simulink model "ModeStatAndRsp"  (R2018b)
settings: Solver=FixedStepDiscrete  StartTime=0.0  StopTime=10.0  FixedStep=0.01  RelTol=1e-3
undefined symbols (not defined in the file): c_RecvL, c_RecvLR, c_RecvR, IfVeSMSeStNumConfig, KeSMSbMdChime2Enable_Val, KeSMSbSRSPosNumConfig_Val, KeSMSuChmReqDurnTm_Val, KeSMSuChmReqIntlTm_Val, KeSMSuRspStatHldTm_Val, MdRspLocal1, MdTp1, ModeNum, PowerMode1, SrcReqTp1, srsconvert
libraries: RspLib x47, simulink x1
(part 8 of 8)

== stateflow chart ModeStatAndRsp/ModeStatAndRsp_Runnable_sys/Subsystem1/Subsystem/Chart ==
  state OffState
    note: /*<REQ_MSM_228>*/
  state SeatBusyChk [function]
    (default) -> (junction 431)
    (junction 431) -> (junction 606) [order 1] : [is6s||is4s]
    (junction 606) -> (junction 777) [order 1] : [is4s]
    (junction 777) -> (junction 779) : {
        | EZEStBsy=1;
        | EZQStBsy=1;
        | LugLStBsy=1;
        | LugRStBsy=1;
        | INTMBsy=1;
        | FamlyLBsy=1;
        | FamlyRBsy=1;
        | INTMRBsy=1;
        | }
    (junction 431) -> (junction 495) [order 2]
    (junction 606) -> (junction 620) [order 2]
    (junction 495) -> (junction 504) [order 1] : [EZQ_En ||VIPL_En||VIPR_En||RecoveryL_En||RecoveryR_En||LugL_En||LugR_En||INTM_En||FAMLY_L_En||FAMLY_R_En||INTMR_En]
    (junction 620) -> (junction 631) [order 1] : [EZQ_En ||VIPL_En||VIPR_En||RecoveryL_En||RecoveryR_En||LugL_En||LugR_En||INTM_En||FAMLY_L_En||FAMLY_R_En||INTMR_En]
    (junction 495) -> (junction 508) [order 2] : {EZEStBsy=0;}
    (junction 504) -> (junction 506) : {EZEStBsy=1;}
    (junction 620) -> (junction 628) [order 2] : {EZEStBsy=0;}
    (junction 631) -> (junction 632) : {EZEStBsy=1;}
    (junction 506) -> (junction 508)
    (junction 632) -> (junction 628)
    (junction 508) -> (junction 511)
    (junction 628) -> (junction 609)
    (junction 609) -> (junction 621) [order 1] : [EZE_En ||VIPL_En||VIPR_En||RecoveryL_En||RecoveryR_En||LugL_En||LugR_En||INTM_En||FAMLY_L_En||FAMLY_R_En||INTMR_En]
    (junction 511) -> (junction 513) [order 1] : [EZE_En ||VIPL_En||VIPR_En||RecoveryL_En||RecoveryR_En||LugL_En||LugR_En||INTM_En||FAMLY_L_En||FAMLY_R_En||INTMR_En]
    (junction 511) -> (junction 517) [order 2] : {EZQStBsy=0;}
    (junction 513) -> (junction 515) : {EZQStBsy=1;}
    (junction 609) -> (junction 624) [order 2] : {EZQStBsy=0;}
    (junction 621) -> (junction 622) : {EZQStBsy=1;}
    (junction 515) -> (junction 517)
    (junction 622) -> (junction 624)
    (junction 517) -> (junction 520)
    (junction 624) -> (junction 619)
    (junction 619) -> (junction 615) [order 1] : [EZE_En||EZQ_En ||RecoveryL_En||LugL_En||INTM_En||FAMLY_L_En||FAMLY_R_En||LugR_En||INTMR_En]
    (junction 520) -> (junction 522) [order 1] : [EZE_En||EZQ_En ||RecoveryL_En||LugL_En||LugR_En||INTM_En||FAMLY_L_En||FAMLY_R_En||INTMR_En]
    (junction 520) -> (junction 526) [order 2] : {VIPLStBsy = 0;}
    (junction 522) -> (junction 524) : {VIPLStBsy = 1;}
    (junction 619) -> (junction 623) [order 2] : {VIPLStBsy = 0;}
    (junction 615) -> (junction 614) : {VIPLStBsy = 1;}
    (junction 524) -> (junction 526)
    (junction 614) -> (junction 623)
    (junction 526) -> (junction 529)
    (junction 623) -> (junction 633)
    (junction 779) -> (junction 781) [order 1] : [LyL_En ||RecoveryL_En||LgrstOpenL_En||LgrstCloseL_En]
    (junction 779) -> (junction 785) [order 2] : {VIPLStBsy = 0;}
    (junction 781) -> (junction 783) : {VIPLStBsy = 1;}
    (junction 529) -> (junction 531) [order 1] : [EZE_En||EZQ_En ||RecoveryR_En||LugL_En||LugR_En||INTM_En||FAMLY_L_En||FAMLY_R_En||INTMR_En]
    (junction 633) -> (junction 608) [order 1] : [EZE_En||EZQ_En ||RecoveryR_En||LugR_En||INTM_En||FAMLY_L_En||FAMLY_R_En||LugL_En||INTMR_En]
    (junction 529) -> (junction 535) [order 2] : {VIPRStBsy = 0;}
    (junction 531) -> (junction 533) : {VIPRStBsy = 1;}
    (junction 633) -> (junction 625) [order 2] : {VIPRStBsy = 0;}
    (junction 608) -> (junction 612) : {VIPRStBsy = 1;}
    (junction 783) -> (junction 785)
    (junction 533) -> (junction 535)
    (junction 612) -> (junction 625)
    (junction 785) -> (junction 788)
    (junction 535) -> (junction 538)
    (junction 625) -> (junction 626)
    (junction 538) -> (junction 540) [order 1] : [EZE_En||EZQ_En ||VIPL_En||LugL_En||LugR_En||INTM_En||FAMLY_L_En||FAMLY_R_En||VIPAll_En||INTMR_En]
    (junction 626) -> (junction 627) [order 1] : [EZE_En||EZQ_En ||VIPL_En||LugL_En||LugR_En||INTM_En||FAMLY_L_En||FAMLY_R_En||VIPR_En||INTMR_En]
    (junction 788) -> (junction 789) [order 1] : [VIPL_En||LyL_En||LgrstOpenL_En||LgrstCloseL_En]
    (junction 538) -> (junction 544) [order 2] : {RecoveryLStBsy = 0;}
    (junction 540) -> (junction 542) : {RecoveryLStBsy = 1;}
    (junction 626) -> (junction 613) [order 2] : {RecoveryLStBsy = 0;}
    (junction 627) -> (junction 630) : {RecoveryLStBsy = 1;}
    (junction 788) -> (junction 793) [order 2] : {RecoveryLStBsy = 0;}
    (junction 789) -> (junction 792) : {RecoveryLStBsy = 1;}
    (junction 792) -> (junction 793)
    (junction 793) -> (junction 797)
    (junction 542) -> (junction 544)
    (junction 630) -> (junction 613)
    (junction 544) -> (junction 547)
    (junction 613) -> (junction 629)
    (junction 797) -> (junction 798) [order 1] : [VIPL_En||RecoveryL_En||LgrstOpenL_En||LgrstCloseL_En]
    (junction 797) -> (junction 802) [order 2] : {LyLBsy = 0;}
    (junction 798) -> (junction 801) : {LyLBsy = 1;}
    (junction 547) -> (junction 549) [order 1] : [EZE_En||EZQ_En ||VIPR_En||LugL_En||LugR_En||INTM_En||FAMLY_L_En||FAMLY_R_En||VIPAll_En||INTMR_En]
    (junction 629) -> (junction 634) [order 1] : [EZE_En||EZQ_En ||VIPR_En||LugL_En||LugR_En||INTM_En||FAMLY_L_En||FAMLY_R_En||VIPAll_En||INTMR_En]
    (junction 547) -> (junction 553) [order 2] : {RecoveryRStBsy = 0;}
    (junction 549) -> (junction 551) : {RecoveryRStBsy = 1;}
    (junction 629) -> (junction 610) [order 2] : {RecoveryRStBsy = 0;}
    (junction 634) -> (junction 611) : {RecoveryRStBsy = 1;}
    (junction 551) -> (junction 553)
    (junction 611) -> (junction 610)
    (junction 801) -> (junction 802)
    (junction 553) -> (junction 556)
    (junction 610) -> (junction 616)
    (junction 802) -> (junction 810)
    (junction 556) -> (junction 558) [order 1] : [EZE_En||EZQ_En ||VIPL_En||VIPR_En||RecoveryL_En||RecoveryR_En||FAMLY_R_En||FAMLY_L_En]
    (junction 616) -> (junction 617) [order 1] : [EZE_En||EZQ_En ||VIPL_En||VIPR_En||RecoveryL_En||RecoveryR_En||FAMLY_R_En||FAMLY_L_En]
    (junction 556) -> (junction 562) [order 2] : {LugLStBsy = 0;}
    (junction 558) -> (junction 560) : {LugLStBsy = 1;}
    (junction 616) -> (junction 618) [order 2] : {LugLStBsy = 0;}
    (junction 617) -> (junction 680) : {LugLStBsy = 1;}
    (junction 810) -> (junction 809) [order 1] : [RecoveryR_En||LyR_En||LgrstOpenR_En||LgrstCloseR_En]
    (junction 810) -> (junction 813) [order 2] : {VIPRStBsy = 0;}
    (junction 809) -> (junction 812) : {VIPRStBsy = 1;}
    (junction 812) -> (junction 813)
    (junction 813) -> (junction 815)
    (junction 560) -> (junction 562)
    (junction 680) -> (junction 618)
    (junction 562) -> (junction 565)
    (junction 618) -> (junction 645)
    (junction 815) -> (junction 816) [order 1] : [VIPR_En||LyR_En||LgrstOpenR_En||LgrstCloseR_En]
    (junction 815) -> (junction 821) [order 2] : {RecoveryRStBsy = 0;}
    (junction 816) -> (junction 822) : {RecoveryRStBsy = 1;}
    (junction 565) -> (junction 567) [order 1] : [EZE_En||EZQ_En ||VIPL_En||VIPR_En||RecoveryL_En||RecoveryR_En||FAMLY_R_En||FAMLY_L_En]
    (junction 645) -> (junction 670) [order 1] : [EZE_En||EZQ_En ||VIPL_En||VIPR_En||RecoveryL_En||RecoveryR_En||FAMLY_R_En||FAMLY_L_En]
    (junction 565) -> (junction 571) [order 2] : {LugRStBsy = 0;}
    (junction 567) -> (junction 569) : {LugRStBsy = 1;}
    (junction 645) -> (junction 675) [order 2] : {LugRStBsy = 0;}
    (junction 670) -> (junction 673) : {LugRStBsy = 1;}
    (junction 822) -> (junction 821)
    (junction 821) -> (junction 824)
    (junction 824) -> (junction 826) [order 1] : [VIPR_En||RecoveryR_En||LgrstOpenR_En||LgrstCloseR_En]
    (junction 569) -> (junction 571)
    (junction 673) -> (junction 675)
    (junction 824) -> (junction 830) [order 2] : {LyRBsy = 0;}
    (junction 826) -> (junction 831) : {LyRBsy = 1;}
    (junction 571) -> (junction 574)
    (junction 675) -> (junction 859)
    (junction 574) -> (junction 833) [order 1] : [EZE_En||EZQ_En ||RecoveryL_En||RecoveryR_En||INTM_En||FAMLY_R_En||VIPL_En||VIPR_En||LugR_En||LugL_En||INTMR_En]
    (junction 859) -> (junction 881) [order 1] : [EZE_En||EZQ_En ||RecoveryL_En||RecoveryR_En||INTM_En||FAMLY_R_En||VIPL_En||VIPR_En||LugR_En||LugL_En||INTMR_En]
    (junction 831) -> (junction 830)
    (junction 574) -> (junction 837) [order 2] : {FamlyLBsy = 0;}
    (junction 833) -> (junction 835) : {FamlyLBsy = 1;}
    (junction 859) -> (junction 858) [order 2] : {FamlyLBsy = 0;}
    (junction 881) -> (junction 879) : {FamlyLBsy = 1;}
    (junction 830) -> (junction 1014)
    (junction 1014) -> (junction 1016) [order 1] : [VIPL_En||RecoveryL_En||LyL_En||LgrstCloseL_En]
    (junction 1014) -> (junction 1020) [order 2] : {LgrstOpenLBsy=0;}
    (junction 1016) -> (junction 1018) : {LgrstOpenLBsy=1;}
    (junction 835) -> (junction 837)
    (junction 879) -> (junction 858)
    (junction 837) -> (junction 841)
    (junction 858) -> (junction 863)
    (junction 841) -> (junction 847) [order 1] : [EZE_En||EZQ_En ||RecoveryL_En||RecoveryR_En||INTM_En||FAMLY_L_En||VIPL_En||VIPR_En||LugL_En||LugR_En||INTMR_En]
    (junction 863) -> (junction 860) [order 1] : [EZE_En||EZQ_En ||RecoveryL_En||RecoveryR_En||INTM_En||FAMLY_L_En||VIPL_En||VIPR_En||LugL_En||LugR_En||INTMR_En]
    (junction 1018) -> (junction 1020)
    (junction 841) -> (junction 840) [order 2] : {FamlyRBsy = 0;}
    (junction 847) -> (junction 845) : {FamlyRBsy = 1;}
    (junction 863) -> (junction 867) [order 2] : {FamlyRBsy = 0;}
    (junction 860) -> (junction 862) : {FamlyRBsy = 1;}
    (junction 1020) -> (junction 1023)
    (junction 1023) -> (junction 1029) [order 1] : [VIPL_En||RecoveryL_En||LyL_En||LgrstOpenL_En]
    (junction 1023) -> (junction 1025) [order 2] : {LgrstCloseLBsy=0;}
    (junction 1029) -> (junction 1030) : {LgrstCloseLBsy=1;}
    (junction 845) -> (junction 840)
    (junction 862) -> (junction 867)
    (junction 840) -> (junction 850)
    (junction 867) -> (junction 869)
    (junction 850) -> (junction 856) [order 1] : [EZE_En||EZQ_En ||RecoveryL_En||RecoveryR_En||FAMLY_L_En||FAMLY_R_En||VIPL_En||VIPR_En||INTMR_En]
    (junction 869) -> (junction 870) [order 1] : [EZE_En||EZQ_En ||RecoveryL_En||RecoveryR_En||FAMLY_L_En||FAMLY_R_En||VIPL_En||VIPR_En||INTMR_En]
    (junction 1030) -> (junction 1025)
    (junction 850) -> (junction 849) [order 2] : {INTMBsy = 0;}
    (junction 856) -> (junction 854) : {INTMBsy = 1;}
    (junction 869) -> (junction 868) [order 2] : {INTMBsy = 0;}
    (junction 870) -> (junction 874) : {INTMBsy = 1;}
    (junction 1025) -> (junction 1040)
    (junction 1040) -> (junction 1034) [order 1] : [VIPR_En||RecoveryR_En||LyR_En||LgrstCloseR_En]
    (junction 1040) -> (junction 1038) [order 2] : {LgrstOpenRBsy=0;}
    (junction 1034) -> (junction 1032) : {LgrstOpenRBsy=1;}
    (junction 854) -> (junction 849)
    (junction 874) -> (junction 868)
    (junction 849) -> (junction 988)
    (junction 868) -> (junction 1002)
    (junction 988) -> (junction 991) [order 1] : [EZE_En||EZQ_En ||RecoveryL_En||RecoveryR_En||FAMLY_L_En||FAMLY_R_En||VIPL_En||VIPR_En||INTM_En]
    (junction 1002) -> (junction 1004) [order 1] : [EZE_En||EZQ_En ||RecoveryL_En||RecoveryR_En||FAMLY_L_En||FAMLY_R_En||VIPL_En||VIPR_En||INTM_En]
    (junction 1032) -> (junction 1038)
    (junction 988) -> (junction 999) [order 2] : {INTMRBsy = 0;}
    (junction 991) -> (junction 997) : {INTMRBsy = 1;}
    (junction 1002) -> (junction 1006) [order 2] : {INTMRBsy = 0;}
    (junction 1004) -> (junction 1008) : {INTMRBsy = 1;}
    (junction 1038) -> (junction 1041)
    (junction 1041) -> (junction 1043) [order 1] : [VIPR_En||RecoveryR_En||LgrstOpenR_En||LyR_En]
    (junction 1041) -> (junction 1047) [order 2] : {LgrstCloseRBsy=0;}
    (junction 1043) -> (junction 1048) : {LgrstCloseRBsy=1;}
    (junction 997) -> (junction 999)
    (junction 1006) -> (junction 997)
    (junction 1008) -> (junction 1006)
    (junction 1047) -> (junction 1008)
    (junction 1048) -> (junction 1047)
    (junction 999) -> (junction 1012)
  note: Easy Entry＞Easy Exit＞VIP＞Recovery＞Luggage。
  state OnState
    en:SeatBusyChk();
    du:SeatBusyChk();
    state EZE [parallel]
      settings: executionOrder=1
      state EZE_entryOngoing
        en:EZE_En = 1;
        en:ModeSrcTpEZE = acsEntyMdSrcTp;
        en:oModeRspEZE = MdRsp_RecallOngoing;
        en:SeatBusyChk();
      state EZEIlde
        en:EZE_En =0;
        en:ModeSrcTpEZE =SrcReqTp1.SrcReqTp_None;
      (default) -> EZEIlde
      EZEIlde -> EZE_entryOngoing : [(acsEntyMdReq)&&EZEStBsy ==0]
      EZE_entryOngoing -> EZEIlde [order 1] : [hasChangedTo(SoftIntAcsEnty,true)]{oModeRspEZE = MdRsp_RecallUnsuccessfully_LocalInterrupt;}
      EZE_entryOngoing -> EZEIlde [order 2] : [hasChangedTo(SwIntAcsEnty,true)]{oModeRspEZE =MdRsp_RecallUnsuccessfully_LocalInterrupt; }
      EZE_entryOngoing -> EZEIlde [order 3] : [hasChangedTo(iIsAcsMdEntryDoneOK,true)]{oModeRspEZE =MdRsp_RecallSuccessfully;}
      EZE_entryOngoing -> EZEIlde [order 4] : [CommExitCondwithSpeed]{oModeRspEZE = MdRsp_RecallUnsuccessfully_Error;}
      EZE_entryOngoing -> EZEIlde [order 5] : [hasChangedTo(iIsAcsMdEntryDoneFailed,true)]{oModeRspEZE = MdRsp_RecallUnsuccessfully_Error;}
    state EZQ [parallel]
      settings: executionOrder=2
      state EZQIlde
        en:EZQ_En =0;
        en:ModeSrcTpEZQ=SrcReqTp1.SrcReqTp_None;
      state EZE_exitOngoing
        en:EZQ_En =1;
        en:ModeSrcTpEZQ = acsExtMdSrcTp;
        en:oModeRspEZQ = MdRsp_RecallOngoing;
        en:SeatBusyChk();
      (default) -> EZQIlde
      EZQIlde -> EZE_exitOngoing : [(acsExtMdReq)&& EZQStBsy == 0]
      EZE_exitOngoing -> EZQIlde [order 1] : [hasChangedTo(SoftIntAcsExt,true)]
          | {oModeRspEZQ = MdRsp_RecallUnsuccessfully_LocalInterrupt;}
      EZE_exitOngoing -> EZQIlde [order 2] : [hasChangedTo(SwIntAcsExt,true)]
          | {oModeRspEZQ = MdRsp_RecallUnsuccessfully_LocalInterrupt;}
      EZE_exitOngoing -> EZQIlde [order 3] : [hasChangedTo(iIsAcsMdExtDoneOK,true)]
          | {oModeRspEZQ = MdRsp_RecallSuccessfully;}
      EZE_exitOngoing -> EZQIlde [order 4] : [CommExitCondwithSpeed]
          | {oModeRspEZQ = MdRsp_RecallUnsuccessfully_Error;}
      EZE_exitOngoing -> EZQIlde [order 5] : [hasChangedTo(iIsAcsMdExtDoneFailed,true)]
          | {oModeRspEZQ = MdRsp_RecallUnsuccessfully_Error;}
    state VIPL [parallel]
      settings: executionOrder=3
      state VIPLIlde
        en:VIPL_En = 0;
        en:ModeSrcTpLtVIP=SrcReqTp1.SrcReqTp_None;
        en:ChkVIPAll();
      state VIPLtOngoing
        en:VIPL_En = 1;
        en:ModeSrcTpALLVIP =AllVipSrcReqTp;
        en:oModeRspLtVIP = MdRsp_RecallOngoing;
        en:SeatBusyChk();
      (default) -> VIPLIlde
      VIPLIlde -> VIPLtOngoing [order 1] : [(AllVipMdReq)&& VIPLStBsy ==0&&VipMdLtAvl==1 ]
          | {VIPAll_En =1;oModeRspVIPALL =MdRsp_RecallOngoing;ModeSrcTpLtVIP=AllVipSrcReqTp;}
      VIPLIlde -> VIPLtOngoing [order 2] : [(LtVipMdReq)&& VIPLStBsy ==0]{ModeSrcTpLtVIP = LtVipSrcReqTp;}
      VIPLtOngoing -> VIPLIlde [order 1] : [hasChangedTo(SoftIntLfVip,true)...
          | ||((hasChangedTo(SoftIntAllVip,true)||hasChangedTo(SwIntAllVip,true))&&VIPAll_En)]{oModeRspLtVIP = MdRsp_RecallUnsuccessfully_LocalInterrupt; }
      VIPLtOngoing -> VIPLIlde [order 2] : [hasChangedTo(SwIntLfVip,true)]{oModeRspLtVIP = MdRsp_RecallUnsuccessfully_LocalInterrupt;}
      VIPLtOngoing -> VIPLIlde [order 3] : [hasChangedTo(iIsLtVipDoneOK,true)]{oModeRspLtVIP = MdRsp_RecallSuccessfully;}
      VIPLtOngoing -> VIPLIlde [order 4] : [CommExitCond]{oModeRspLtVIP = MdRsp_RecallUnsuccessfully_Error;}
      VIPLtOngoing -> VIPLIlde [order 5] : [hasChangedTo(iIsLtVipDoneFailed,true)]{oModeRspLtVIP = MdRsp_RecallUnsuccessfully_Error;}
    state VIPR [parallel]
      settings: executionOrder=4
      state VIPRtOngoing
        en:VIPR_En = 1;
        en:ModeSrcTpALLVIP =AllVipSrcReqTp;
        en:oModeRspRtVIP = MdRsp_RecallOngoing;
        en:SeatBusyChk();
      state VIPRIdle
        en:VIPR_En = 0;
        en:ModeSrcTpRtVIP=SrcReqTp1.SrcReqTp_None;
        en:ChkVIPAll();
      (default) -> VIPRIdle
      VIPRIdle -> VIPRtOngoing [order 1] : [(AllVipMdReq)&&VIPRStBsy ==0&&VipMdRtAvl==1 ]
          | {VIPAll_En = 1;oModeRspVIPALL =MdRsp_RecallOngoing;ModeSrcTpRtVIP=AllVipSrcReqTp;}
      VIPRIdle -> VIPRtOngoing [order 2] : [(RtVipMdReq)&&VIPRStBsy ==0]{ModeSrcTpRtVIP = RtVipSrcReqTp;}
      VIPRtOngoing -> VIPRIdle [order 1] : [hasChangedTo(SoftIntRtVip,true)...
          | ||((hasChangedTo(SoftIntAllVip,true)||hasChangedTo(SwIntAllVip,true))&&VIPAll_En)]{oModeRspRtVIP = MdRsp_RecallUnsuccessfully_LocalInterrupt;}
      VIPRtOngoing -> VIPRIdle [order 2] : [hasChangedTo(SwIntRtVip,true)]{oModeRspRtVIP = MdRsp_RecallUnsuccessfully_LocalInterrupt; }
      VIPRtOngoing -> VIPRIdle [order 3] : [hasChangedTo(iIsRtVipDoneOK,true)]{oModeRspRtVIP = MdRsp_RecallSuccessfully}
      VIPRtOngoing -> VIPRIdle [order 4] : [CommExitCond]{oModeRspRtVIP = MdRsp_RecallUnsuccessfully_Error;}
      VIPRtOngoing -> VIPRIdle [order 5] : [hasChangedTo(iIsRtVipDoneFailed,true)]{oModeRspRtVIP = MdRsp_RecallUnsuccessfully_Error}
    state RecoveryL [parallel]
      settings: executionOrder=5
      state RecoveryLtOngoing
        en:RecoveryL_En =1;
        en:ModeSrcTpLtRecovery = LtRcvySrcReqTp;
        en:oModeRspLtRecovery = MdRsp_RecallOngoing;
        en:SeatBusyChk();
      state RecoveryLIlde
        en:RecoveryL_En = 0;
        en:ModeSrcTpLtRecovery=SrcReqTp1.SrcReqTp_None;
      (default) -> RecoveryLIlde
      RecoveryLIlde -> RecoveryLtOngoing : [(LtRcvyMdReq)&&RecoveryLStBsy == 0]
      RecoveryLtOngoing -> RecoveryLIlde [order 1] : [hasChangedTo(SoftIntLfRcvy,true)]
          | {oModeRspLtRecovery = MdRsp_RecallUnsuccessfully_LocalInterrupt;}
      RecoveryLtOngoing -> RecoveryLIlde [order 2] : [hasChangedTo(SwIntLfRcvy,true)]
          | {oModeRspLtRecovery = MdRsp_RecallUnsuccessfully_LocalInterrupt;}
      RecoveryLtOngoing -> RecoveryLIlde [order 3] : [hasChangedTo(iIsLtRecoveryDoneOK,true) ]
          | {oModeRspLtRecovery = MdRsp_RecallSuccessfully;}
      RecoveryLtOngoing -> RecoveryLIlde [order 4] : [CommExitCond]{oModeRspLtRecovery = MdRsp_RecallUnsuccessfully_Error;}
      RecoveryLtOngoing -> RecoveryLIlde [order 5] : [hasChangedTo(iIsLtRecoveryDoneFailed,true)]
          | {oModeRspLtRecovery = MdRsp_RecallUnsuccessfully_Error;}
    state RecoveryR [parallel]
      settings: executionOrder=6
      state RecoveryRIdle
        en:RecoveryR_En =0;
        en:ModeSrcTpRtRecovery=SrcReqTp1.SrcReqTp_None;
      state RecoveryRtOngoing
        en:RecoveryR_En = 1;
        en:ModeSrcTpRtRecovery = RtRcvySrcReqTp;
        en:oModeRspRtRecovery = MdRsp_RecallOngoing;
        en:SeatBusyChk();
      (default) -> RecoveryRIdle
      RecoveryRIdle -> RecoveryRtOngoing : [(RtRcvyMdReq)&& RecoveryRStBsy ==0]
      RecoveryRtOngoing -> RecoveryRIdle [order 1] : [hasChangedTo(SoftIntRtRcvy,true)]{oModeRspRtRecovery = MdRsp_RecallUnsuccessfully_LocalInterrupt;}
      RecoveryRtOngoing -> RecoveryRIdle [order 2] : [hasChangedTo(SwIntRtRcvy,true)]{oModeRspRtRecovery = MdRsp_RecallUnsuccessfully_LocalInterrupt;}
      RecoveryRtOngoing -> RecoveryRIdle [order 3] : [hasChangedTo(iIsRtRecoveryDoneOK,true)]{oModeRspRtRecovery = MdRsp_RecallSuccessfully;}
      RecoveryRtOngoing -> RecoveryRIdle [order 4] : [CommExitCond]{oModeRspRtRecovery = MdRsp_RecallUnsuccessfully_Error;}
      RecoveryRtOngoing -> RecoveryRIdle [order 5] : [hasChangedTo(iIsRtRecoveryDoneFailed,true)]{oModeRspRtRecovery = MdRsp_RecallUnsuccessfully_Error;}
    state FamlyL [parallel]
      settings: executionOrder=7
      state FamlyLOngoing
        en:FAMLY_L_En = 1;
        en:ModeSrcTpLfFamly = LfFamlySrcReqTp;
        en:oModeRspLfFamly = MdRsp_RecallOngoing;
        en:SeatBusyChk();
      state FamlyLIdle
        en:FAMLY_L_En =0;
        en:ModeSrcTpLfFamly=SrcReqTp1.SrcReqTp_None;
      (default) -> FamlyLIdle
      FamlyLIdle -> FamlyLOngoing : [(LfFamlyMdReq)&&FamlyLBsy ==0]
      FamlyLOngoing -> FamlyLIdle [order 1] : [hasChangedTo(SoftIntLfFamly,true)]
          | {oModeRspLfFamly = MdRsp_RecallUnsuccessfully_LocalInterrupt;}
      FamlyLOngoing -> FamlyLIdle [order 2] : [hasChangedTo(SwIntLfFamly,true)]
          | {oModeRspLfFamly = MdRsp_RecallUnsuccessfully_LocalInterrupt; }
      FamlyLOngoing -> FamlyLIdle [order 3] : [hasChangedTo(isFamlyLDoneOK,true)]{oModeRspLfFamly = MdRsp_RecallSuccessfully;}
      FamlyLOngoing -> FamlyLIdle [order 4] : [CommExitCond]{oModeRspLfFamly = MdRsp_RecallUnsuccessfully_Error;}
      FamlyLOngoing -> FamlyLIdle [order 5] : [hasChangedTo(isFamlyLDoneFailed,true)]{oModeRspLfFamly = MdRsp_RecallUnsuccessfully_Error;}
    state FamlyR [parallel]
      settings: executionOrder=8
      state FamlyROngoing
        en:FAMLY_R_En = 1;
        en:ModeSrcTpRtFamly = RtFamlySrcReqTp;
        en:oModeRspRtFamly = MdRsp_RecallOngoing;
        en:SeatBusyChk();
      state FamlyRIdle
        en:FAMLY_R_En =0;
        en:ModeSrcTpRtFamly=SrcReqTp1.SrcReqTp_None;
      (default) -> FamlyRIdle
      FamlyRIdle -> FamlyROngoing : [(RtFamlyMdReq)&&FamlyRBsy ==0]
      FamlyROngoing -> FamlyRIdle [order 1] : [hasChangedTo(SoftIntRtFamly,true)]
          | {oModeRspRtFamly = MdRsp_RecallUnsuccessfully_LocalInterrupt;}
      FamlyROngoing -> FamlyRIdle [order 2] : [hasChangedTo(SwIntRtFamly,true)]
          | {oModeRspRtFamly = MdRsp_RecallUnsuccessfully_LocalInterrupt; }
      FamlyROngoing -> FamlyRIdle [order 3] : [hasChangedTo(isFamlyRDoneOK,true)]{oModeRspRtFamly = MdRsp_RecallSuccessfully;}
      FamlyROngoing -> FamlyRIdle [order 4] : [CommExitCond]{oModeRspRtFamly = MdRsp_RecallUnsuccessfully_Error;}
      FamlyROngoing -> FamlyRIdle [order 5] : [hasChangedTo(isFamlyRDoneFailed,true)]{oModeRspRtFamly = MdRsp_RecallUnsuccessfully_Error;}
    state INTM [parallel]
      settings: executionOrder=9
      state INTMOngoing
        en:INTM_En = 1;
        en:ModeSrcTpINTM = INTMSrcReqTp;
        en:oModeRspINTM = MdRsp_RecallOngoing;
        en:SeatBusyChk();
      state INTMIdle
        en:INTM_En =0;
        en:ModeSrcTpINTM=SrcReqTp1.SrcReqTp_None;
      (default) -> INTMIdle
      INTMIdle -> INTMOngoing : [(INTMMdReq)&&INTMBsy ==0]
      INTMOngoing -> INTMIdle [order 1] : [hasChangedTo(SoftIntINTM,true)]
          | {oModeRspINTM = MdRsp_RecallUnsuccessfully_LocalInterrupt;}
      INTMOngoing -> INTMIdle [order 2] : [hasChangedTo(SwIntINTM,true)]
          | {oModeRspINTM = MdRsp_RecallUnsuccessfully_LocalInterrupt; }
      INTMOngoing -> INTMIdle [order 3] : [hasChangedTo(isINTMDoneOK,true)]{oModeRspINTM = MdRsp_RecallSuccessfully;}
      INTMOngoing -> INTMIdle [order 4] : [CommExitCond]{oModeRspINTM = MdRsp_RecallUnsuccessfully_Error;}
      INTMOngoing -> INTMIdle [order 5] : [hasChangedTo(isINTMDoneFailed,true)]{oModeRspINTM = MdRsp_RecallUnsuccessfully_Error;}
    state INTMR [parallel]
      settings: executionOrder=10
      state INTMROngoing
        en:INTMR_En = 1;
        en:ModeSrcTpINTMR = INTMRSrcReqTp;
        en:oModeRspINTMR = MdRsp_RecallOngoing;
        en:SeatBusyChk();
      state INTMRIdle
        en:INTMR_En =0;
        en:ModeSrcTpINTMR=SrcReqTp1.SrcReqTp_None;
      (default) -> INTMRIdle
      INTMRIdle -> INTMROngoing : [(INTMRMdReq)&&INTMRBsy ==0]
      INTMROngoing -> INTMRIdle [order 1] : [hasChangedTo(SoftIntINTMR,true)]
          | {oModeRspINTMR = MdRsp_RecallUnsuccessfully_LocalInterrupt;}
      INTMROngoing -> INTMRIdle [order 2] : [hasChangedTo(SwIntINTMR,true)]
          | {oModeRspINTMR = MdRsp_RecallUnsuccessfully_LocalInterrupt; }
      INTMROngoing -> INTMRIdle [order 3] : [hasChangedTo(isINTMRDoneOK,true)]{oModeRspINTMR = MdRsp_RecallSuccessfully;}
      INTMROngoing -> INTMRIdle [order 4] : [CommExitCond]{oModeRspINTMR = MdRsp_RecallUnsuccessfully_Error;}
      INTMROngoing -> INTMRIdle [order 5] : [hasChangedTo(isINTMRDoneFailed,true)]{oModeRspINTMR = MdRsp_RecallUnsuccessfully_Error;}
    state LugL [parallel]
      settings: executionOrder=11
      state LugLIlde
        en:LugL_En =0;
        en:ModeSrcTpLtLug =SrcReqTp1.SrcReqTp_None;
        en:ChkLugAll();
      state LugLtOngoing
        en:LugL_En =1;
        en:ModeSrcTpAllLug = AllLugSrcReqTp;
        en:oModeRspLtLug = MdRsp_RecallOngoing;
        en:SeatBusyChk();
      (default) -> LugLIlde
      LugLIlde -> LugLtOngoing [order 1] : [(AllLugMdReq)&&LugLStBsy ==0&&LugMdLtAvl ==1]
          | {LugAll_En=1;oModeRspLugALL=MdRsp_RecallOngoing;ModeSrcTpLtLug = AllLugSrcReqTp;}
      LugLIlde -> LugLtOngoing [order 2] : [(LtLugMdReq)&&LugLStBsy ==0]{ModeSrcTpLtLug = LtLugSrcReqTp;}
      LugLtOngoing -> LugLIlde [order 1] : [hasChangedTo(SoftIntLfLug,true)...
          | ||(hasChangedTo(SoftIntAllLug,true)&&LugAll_En)]
          | {oModeRspLtLug = MdRsp_RecallUnsuccessfully_LocalInterrupt;}
      LugLtOngoing -> LugLIlde [order 2] : [hasChangedTo(SwIntLfLug,true)...
          | ||(hasChangedTo(SwIntAllLug,true)&&LugAll_En)]
          | {oModeRspLtLug = MdRsp_RecallUnsuccessfully_LocalInterrupt;}
      LugLtOngoing -> LugLIlde [order 3] : [hasChangedTo(iIsLtLugDoneOK,true) ]
          | {oModeRspLtLug = MdRsp_RecallSuccessfully;}/*<REQ_MSM_420>*/
      LugLtOngoing -> LugLIlde [order 4] : [CommExitCondwithSpeed]{oModeRspLtLug = MdRsp_RecallUnsuccessfully_Error;}/*<REQ_MSM_435>*/
      LugLtOngoing -> LugLIlde [order 5] : [hasChangedTo(iIsLtLugDoneFailed,true)]
          | {oModeRspLtLug = MdRsp_RecallUnsuccessfully_Error;}/*<REQ_MSM_420>*/
    state LugR [parallel]
      settings: executionOrder=12
      state LugRtOngoing
        en:LugR_En = 1;
        en:ModeSrcTpAllLug = AllLugSrcReqTp;
        en:oModeRspRtLug = MdRsp_RecallOngoing;
        en:SeatBusyChk();
      state LugRIdle
        en:LugR_En =0;
        en:ModeSrcTpRtLug =SrcReqTp1.SrcReqTp_None;
        en:ChkLugAll();
      (default) -> LugRIdle
      LugRIdle -> LugRtOngoing [order 1] : [(AllLugMdReq)&&LugRStBsy ==0&&LugMdRtAvl==1]
          | {LugAll_En=1;oModeRspLugALL=MdRsp_RecallOngoing;ModeSrcTpRtLug = AllLugSrcReqTp;}
      LugRIdle -> LugRtOngoing [order 2] : [(RtLugMdReq)&&LugRStBsy ==0]{ModeSrcTpRtLug = RtLugSrcReqTp;}
      LugRtOngoing -> LugRIdle [order 1] : [hasChangedTo(SoftIntRtLug,true)...
          | ||(hasChangedTo(SoftIntAllLug,true)&&LugAll_En)]{oModeRspRtLug = MdRsp_RecallUnsuccessfully_LocalInterrupt;}
      LugRtOngoing -> LugRIdle [order 2] : [hasChangedTo(SwIntRtLug,true)...
          | ||(hasChangedTo(SwIntAllLug,true)&&LugAll_En)]{oModeRspRtLug = MdRsp_RecallUnsuccessfully_LocalInterrupt; }
      LugRtOngoing -> LugRIdle [order 3] : [hasChangedTo(iIsRtLugDoneOK,true)]{oModeRspRtLug = MdRsp_RecallSuccessfully;}
      LugRtOngoing -> LugRIdle [order 4] : [CommExitCondwithSpeed]{oModeRspRtLug = MdRsp_RecallUnsuccessfully_Error;}
      LugRtOngoing -> LugRIdle [order 5] : [hasChangedTo(iIsRtLugDoneFailed,true)]{oModeRspRtLug = MdRsp_RecallUnsuccessfully_Error;}
    state LyL [parallel]
      settings: executionOrder=13
      state LyLOngoing
        en:LyL_En = 1;
        en:ModeSrcTpLfLy = LfLySrcReqTp;
        en:oModeRspLfLy = MdRsp_RecallOngoing;
        en:SeatBusyChk();
      state LyLIdle
        en:LyL_En =0;
        en:ModeSrcTpLfLy=SrcReqTp1.SrcReqTp_None;
      (default) -> LyLIdle
      LyLIdle -> LyLOngoing : [(LfLyMdReq)&&LyLBsy ==0]
      LyLOngoing -> LyLIdle [order 1] : [hasChangedTo(SoftIntLfLy,true)]
          | {oModeRspLfLy = MdRsp_RecallUnsuccessfully_LocalInterrupt;}
      LyLOngoing -> LyLIdle [order 2] : [hasChangedTo(SwIntLfLy,true)]
          | {oModeRspLfLy = MdRsp_RecallUnsuccessfully_LocalInterrupt; }
      LyLOngoing -> LyLIdle [order 3] : [hasChangedTo(isLfLyDoneOK,true)]{oModeRspLfLy = MdRsp_RecallSuccessfully;}
      LyLOngoing -> LyLIdle [order 4] : [CommExitCond]{oModeRspLfLy = MdRsp_RecallUnsuccessfully_Error;}
      LyLOngoing -> LyLIdle [order 5] : [hasChangedTo(isLfLyDoneFailed,true)]{oModeRspLfLy = MdRsp_RecallUnsuccessfully_Error;}
    state LyR [parallel]
      settings: executionOrder=14
      state LyROngoing
        en:LyR_En = 1;
        en:ModeSrcTpRtLy = RtLySrcReqTp;
        en:oModeRspRtLy = MdRsp_RecallOngoing;
        en:SeatBusyChk();
      state LyRIdle
        en:LyR_En =0;
        en:ModeSrcTpRtLy=SrcReqTp1.SrcReqTp_None;
      (default) -> LyRIdle
      LyRIdle -> LyROngoing : [(RtLyMdReq)&&LyRBsy ==0]
      LyROngoing -> LyRIdle [order 1] : [hasChangedTo(SoftIntRtLy,true)]
          | {oModeRspRtLy = MdRsp_RecallUnsuccessfully_LocalInterrupt;}
      LyROngoing -> LyRIdle [order 2] : [hasChangedTo(SwIntRtLy,true)]
          | {oModeRspRtLy = MdRsp_RecallUnsuccessfully_LocalInterrupt; }
      LyROngoing -> LyRIdle [order 3] : [hasChangedTo(isRtLyDoneOK,true)]{oModeRspRtLy = MdRsp_RecallSuccessfully;}
      LyROngoing -> LyRIdle [order 4] : [CommExitCond]{oModeRspRtLy = MdRsp_RecallUnsuccessfully_Error;}
      LyROngoing -> LyRIdle [order 5] : [hasChangedTo(isRtLyDoneFailed,true)]{oModeRspRtLy = MdRsp_RecallUnsuccessfully_Error;}
    state LgrstOpenL [parallel]
      settings: executionOrder=15
      state LgrstOpenLOngoing
        en:LgrstOpenL_En = 1;
        en:ModeSrcTpLgrstOpenL = LgrstOpenLtSrcReqTp;
        en:oModeRspLgrstOpenL = MdRsp_RecallOngoing;
        en:SeatBusyChk();
      state LgrstOpenLIdle
        en:LgrstOpenL_En =0;
        en:ModeSrcTpLgrstOpenL=SrcReqTp1.SrcReqTp_None;
      (default) -> LgrstOpenLIdle
      LgrstOpenLIdle -> LgrstOpenLOngoing : [(LgrstOpenLtMdReq)&&LgrstOpenLBsy ==0]
      LgrstOpenLOngoing -> LgrstOpenLIdle [order 1] : [hasChangedTo(SoftIntLgrstOpenLt,true)]
          | {oModeRspLgrstOpenL = MdRsp_RecallUnsuccessfully_LocalInterrupt;}
      LgrstOpenLOngoing -> LgrstOpenLIdle [order 2] : [hasChangedTo(SwIntLgrstOpenLt,true)]
          | {oModeRspLgrstOpenL = MdRsp_RecallUnsuccessfully_LocalInterrupt; }
      LgrstOpenLOngoing -> LgrstOpenLIdle [order 3] : [hasChangedTo(isLgrstOpenLDoneOK,true)]{oModeRspLgrstOpenL = MdRsp_RecallSuccessfully;}
      LgrstOpenLOngoing -> LgrstOpenLIdle [order 4] : [CommExitCond]{oModeRspLgrstOpenL = MdRsp_RecallUnsuccessfully_Error;}
      LgrstOpenLOngoing -> LgrstOpenLIdle [order 5] : [hasChangedTo(isLgrstOpenLDoneFailed,true)]{oModeRspLgrstOpenL = MdRsp_RecallUnsuccessfully_Error;}
    state LgrstOpenR [parallel]
      settings: executionOrder=16
      state LgrstOpenROngoing
        en:LgrstOpenR_En = 1;
        en:ModeSrcTpLgrstOpenR = LgrstOpenRtSrcReqTp;
        en:oModeRspLgrstOpenR = MdRsp_RecallOngoing;
        en:SeatBusyChk();
      state LgrstOpenRIdle
        en:LgrstOpenR_En =0;
        en:ModeSrcTpLgrstOpenR=SrcReqTp1.SrcReqTp_None;
      (default) -> LgrstOpenRIdle
      LgrstOpenRIdle -> LgrstOpenROngoing : [(LgrstOpenRtMdReq)&&LgrstOpenRBsy ==0]
      LgrstOpenROngoing -> LgrstOpenRIdle [order 1] : [hasChangedTo(SoftIntLgrstOpenRt,true)]
          | {oModeRspLgrstOpenR = MdRsp_RecallUnsuccessfully_LocalInterrupt;}
      LgrstOpenROngoing -> LgrstOpenRIdle [order 2] : [hasChangedTo(SwIntLgrstOpenRt,true)]
          | {oModeRspLgrstOpenR = MdRsp_RecallUnsuccessfully_LocalInterrupt; }
      LgrstOpenROngoing -> LgrstOpenRIdle [order 3] : [hasChangedTo(isLgrstOpenRDoneOK,true)]{oModeRspLgrstOpenR = MdRsp_RecallSuccessfully;}
      LgrstOpenROngoing -> LgrstOpenRIdle [order 4] : [CommExitCond]{oModeRspLgrstOpenR = MdRsp_RecallUnsuccessfully_Error;}
      LgrstOpenROngoing -> LgrstOpenRIdle [order 5] : [hasChangedTo(isLgrstOpenRDoneFailed,true)]{oModeRspLgrstOpenR = MdRsp_RecallUnsuccessfully_Error;}
    state LgrstCloseL [parallel]
      settings: executionOrder=17
      state LgrstCloseLOngoing
        en:LgrstCloseL_En = 1;
        en:ModeSrcTpLgrstCloseL = LgrstCloseLtSrcReqTp;
        en:oModeRspLgrstCloseL = MdRsp_RecallOngoing;
        en:SeatBusyChk();
      state LgrstCloseLIdle
        en:LgrstCloseL_En =0;
        en:ModeSrcTpLgrstCloseL=SrcReqTp1.SrcReqTp_None;
      (default) -> LgrstCloseLIdle
      LgrstCloseLIdle -> LgrstCloseLOngoing : [(LgrstCloseLtMdReq)&&LgrstCloseLBsy ==0]
      LgrstCloseLOngoing -> LgrstCloseLIdle [order 1] : [hasChangedTo(SoftIntLgrstCloseLt,true)]
          | {oModeRspLgrstCloseL = MdRsp_RecallUnsuccessfully_LocalInterrupt;}
      LgrstCloseLOngoing -> LgrstCloseLIdle [order 2] : [hasChangedTo(SwIntLgrstCloseLt,true)]
          | {oModeRspLgrstCloseL = MdRsp_RecallUnsuccessfully_LocalInterrupt; }
      LgrstCloseLOngoing -> LgrstCloseLIdle [order 3] : [hasChangedTo(isLgrstCloseLDoneOK,true)]{oModeRspLgrstCloseL = MdRsp_RecallSuccessfully;}
      LgrstCloseLOngoing -> LgrstCloseLIdle [order 4] : [CommExitCond]{oModeRspLgrstCloseL = MdRsp_RecallUnsuccessfully_Error;}
      LgrstCloseLOngoing -> LgrstCloseLIdle [order 5] : [hasChangedTo(isLgrstCloseLDoneFailed,true)]{oModeRspLgrstCloseL = MdRsp_RecallUnsuccessfully_Error;}
    state LgrstCloseR [parallel]
      settings: executionOrder=18
      state LgrstCloseROngoing
        en:LgrstCloseR_En = 1;
        en:ModeSrcTpLgrstCloseR = LgrstCloseRtSrcReqTp;
        en:oModeRspLgrstCloseR = MdRsp_RecallOngoing;
        en:SeatBusyChk();
      state LgrstCloseRIdle
        en:LgrstCloseR_En =0;
        en:ModeSrcTpLgrstCloseR=SrcReqTp1.SrcReqTp_None;
      (default) -> LgrstCloseRIdle
      LgrstCloseRIdle -> LgrstCloseROngoing : [(LgrstCloseRtMdReq)&&LgrstCloseRBsy ==0]
      LgrstCloseROngoing -> LgrstCloseRIdle [order 1] : [hasChangedTo(SoftIntLgrstCloseRt,true)]
          | {oModeRspLgrstCloseR = MdRsp_RecallUnsuccessfully_LocalInterrupt;}
      LgrstCloseROngoing -> LgrstCloseRIdle [order 2] : [hasChangedTo(SwIntLgrstCloseRt,true)]
          | {oModeRspLgrstCloseR = MdRsp_RecallUnsuccessfully_LocalInterrupt; }
      LgrstCloseROngoing -> LgrstCloseRIdle [order 3] : [hasChangedTo(isLgrstCloseRDoneOK,true)]{oModeRspLgrstCloseR = MdRsp_RecallSuccessfully;}
      LgrstCloseROngoing -> LgrstCloseRIdle [order 4] : [CommExitCond]{oModeRspLgrstCloseR = MdRsp_RecallUnsuccessfully_Error;}
      LgrstCloseROngoing -> LgrstCloseRIdle [order 5] : [hasChangedTo(isLgrstCloseRDoneFailed,true)]{oModeRspLgrstCloseR = MdRsp_RecallUnsuccessfully_Error;}
  state ChkVIPAll [function]
    (default) -> (junction 895)
    (junction 895) -> (junction 897) [order 1] : [VIPAll_En ==1&&VIPL_En==0&&VIPR_En==0]
    (junction 897) -> (junction 904) [order 1] : [VipMdLtAvl==VipMdRtAvl && oModeRspLtVIP ==oModeRspRtVIP]
    (junction 895) -> (junction 901) [order 2]
    (junction 897) -> (junction 899) [order 2] : {
        | VIPAll_En=0;
        | oModeRspVIPALL =MdRsp_RecallUnsuccessfully_Error;
        | ModeSrcTpALLVIP=SrcReqTp1.SrcReqTp_None;
        | }
    (junction 904) -> (junction 906) : {
        | VIPAll_En = 0;
        | oModeRspVIPALL =oModeRspLtVIP;
        | ModeSrcTpALLVIP =  SrcReqTp1.SrcReqTp_None;
        | }
    (junction 899) -> (junction 901)
    (junction 906) -> (junction 899)
  state ChkLugAll [function]
    (default) -> (junction 910)
    (junction 910) -> (junction 911) [order 1] : [LugAll_En ==1&&LugL_En==0&&LugR_En==0]
    (junction 911) -> (junction 912) [order 1] : [LugMdLtAvl ==LugMdRtAvl && oModeRspLtLug ==oModeRspRtLug]
    (junction 910) -> (junction 913) [order 2]
    (junction 911) -> (junction 914) [order 2] : {
        | LugAll_En=0;
        | oModeRspLugALL =MdRsp_RecallUnsuccessfully_Error;
        | ModeSrcTpAllLug=SrcReqTp1.SrcReqTp_None;
        | }
    (junction 912) -> (junction 915) : {
        | LugAll_En = 0;
        | oModeRspLugALL =oModeRspLtLug;
        | ModeSrcTpAllLug =  SrcReqTp1.SrcReqTp_None;
        | }
    (junction 914) -> (junction 913)
    (junction 915) -> (junction 914)
  (default) -> OffState
  OffState -> OnState : [CommCond]
  OnState -> OffState : [!CommCond&&modestate32==0]
  data: acsExtMdReq input boolean; acsEntyMdReq input boolean; LtVipMdReq input boolean; RtVipMdReq input boolean; AllVipMdReq input boolean; LtLugMdReq input boolean; RtLugMdReq input boolean; AllLugMdReq input boolean; LtRcvyMdReq input boolean; RtRcvyMdReq input boolean; CommCond input boolean; CommExitCond input boolean; CommExitCondwithSpeed input boolean; iIsAcsMdEntryDoneOK input boolean; iIsAcsMdExtDoneOK input boolean; iIsLtLugDoneOK input boolean; iIsLtRecoveryDoneOK input boolean; iIsLtVipDoneOK input boolean; iIsRtLugDoneOK input boolean; iIsRtRecoveryDoneOK input boolean; iIsRtVipDoneOK input boolean; iIsAcsMdEntryDoneFailed input boolean; iIsAcsMdExtDoneFailed input boolean; iIsLtLugDoneFailed input boolean; iIsLtRecoveryDoneFailed input boolean; iIsLtVipDoneFailed input boolean; iIsRtLugDoneFailed input boolean; iIsRtRecoveryDoneFailed input boolean; iIsRtVipDoneFailed input boolean; SwIntAcsEnty input boolean; SwIntAcsExt input boolean; SwIntLfVip input boolean; SwIntRtVip input boolean; SwIntLfLug input boolean; SwIntRtLug input boolean; SwIntLfRcvy input boolean; SwIntRtRcvy input boolean; SwIntAllLug input boolean; SoftIntAcsExt input boolean; SoftIntAcsEnty input boolean; SoftIntLfVip input boolean; SoftIntRtVip input boolean; SoftIntLfLug input boolean; SoftIntRtLug input boolean; SoftIntLfRcvy input boolean; SoftIntRtRcvy input boolean; SoftIntAllVip input boolean; SoftIntAllLug input boolean; acsExtMdSrcTp input Enum: SrcReqTp1; acsEntyMdSrcTp input Enum: SrcReqTp1; LtVipSrcReqTp input Enum: SrcReqTp1; RtVipSrcReqTp input Enum: SrcReqTp1; LtLugSrcReqTp input Enum: SrcReqTp1; RtLugSrcReqTp input Enum: SrcReqTp1; LtRcvySrcReqTp input Enum: SrcReqTp1; RtRcvySrcReqTp input Enum: SrcReqTp1; AllLugSrcReqTp input Enum: SrcReqTp1; tmpsrc local Enum: SrcReqTp1; LugAlltmp local boolean; VipAllTmp local boolean; EZE_En output boolean; VIPAll_En output boolean; LugAll_En output boolean; EZQ_En output boolean; INTM_En output boolean; FAMLY_R_En output boolean; FAMLY_L_En output boolean; LugL_En output boolean; LugR_En output boolean; VIPL_En output boolean; RecoveryL_En output boolean; VIPR_En output boolean; RecoveryR_En output boolean; LyL_En output boolean; LyR_En output boolean; LgrstOpenL_En output boolean; LgrstCloseL_En output boolean; LgrstOpenR_En output boolean; LgrstCloseR_En output boolean; INTMR_En output boolean; DrvBsy local boolean; PassBsy local boolean; L2Bsy local boolean; R2Bsy local boolean; L3Bsy local boolean; R3Bsy local boolean; ModeSrcTpAllLug output Enum: SrcReqTp1; ModeSrcTpEZE output Enum: SrcReqTp1; ModeSrcTpEZQ output Enum: SrcReqTp1; ModeSrcTpLtLug output Enum: SrcReqTp1; ModeSrcTpLtRecovery output Enum: SrcReqTp1; ModeSrcTpLtVIP output Enum: SrcReqTp1; ModeSrcTpRtLug output Enum: SrcReqTp1; ModeSrcTpRtRecovery output Enum: SrcReqTp1; ModeSrcTpRtVIP output Enum: SrcReqTp1; oModeRspEZE output Enum: MdRspLocal1; oModeRspEZQ output Enum: MdRspLocal1; oModeRspLtLug output Enum: MdRspLocal1; oModeRspLtRecovery output Enum: MdRspLocal1; oModeRspLtVIP output Enum: MdRspLocal1; oModeRspRtLug output Enum: MdRspLocal1; oModeRspRtRecovery output Enum: MdRspLocal1; oModeRspRtVIP output Enum: MdRspLocal1; oModeRspVIPALL output Enum: MdRspLocal1; oModeRspLugALL output Enum: MdRspLocal1; modestate32 input uint32; INTMMdReq input boolean; LfFamlyMdReq input boolean; LfLyMdReq input boolean; RtFamlyMdReq input boolean; RtLyMdReq input boolean; SoftIntINTM input boolean; SoftIntLfFamly input boolean; SoftIntLfLy input boolean; SoftIntRtFamly input boolean; SoftIntRtLy input boolean; SwIntINTM input boolean; SwIntLfFamly input boolean; SwIntLfLy input boolean; SwIntRtFamly input boolean; SwIntRtLy input boolean; isINTMDoneOK input boolean; isFamlyLDoneOK input boolean; isFamlyRDoneOK input boolean; isLfLyDoneOK input boolean; isRtLyDoneOK input boolean; isINTMDoneFailed input boolean; isFamlyLDoneFailed input boolean; isFamlyRDoneFailed input boolean; isLfLyDoneFailed input boolean; isRtLyDoneFailed input boolean; INTMSrcReqTp input Enum: SrcReqTp1; LfFamlySrcReqTp input Enum: SrcReqTp1; LfLySrcReqTp input Enum: SrcReqTp1; RtFamlySrcReqTp input Enum: SrcReqTp1; RtLySrcReqTp input Enum: SrcReqTp1; ModeSrcTpINTM output Enum: SrcReqTp1; ModeSrcTpLfFamly output Enum: SrcReqTp1; ModeSrcTpLfLy output Enum: SrcReqTp1; ModeSrcTpRtFamly output Enum: SrcReqTp1; ModeSrcTpRtLy output Enum: SrcReqTp1; oModeRspINTM output Enum: MdRspLocal1; oModeRspLfFamly output Enum: MdRspLocal1; oModeRspLfLy output Enum: MdRspLocal1; oModeRspRtFamly output Enum: MdRspLocal1; oModeRspRtLy output Enum: MdRspLocal1; AllVipSrcReqTp input Enum: SrcReqTp1; ModeSrcTpALLVIP output Enum: SrcReqTp1; EZEStBsy output boolean; EZQStBsy output boolean; VIPLStBsy output boolean; VIPRStBsy output boolean; RecoveryLStBsy output boolean; RecoveryRStBsy output boolean; LugLStBsy output boolean; LugRStBsy output boolean; FamlyLBsy output boolean; FamlyRBsy output boolean; INTMBsy output boolean; LyLBsy output boolean; LyRBsy output boolean; LugMdLtAvl input boolean; LugMdRtAvl input boolean; VipMdLtAvl input boolean; VipMdRtAvl input boolean; SwIntAllVip input boolean; INTMRMdReq input boolean; LgrstCloseLtMdReq input boolean; LgrstCloseRtMdReq input boolean; LgrstOpenLtMdReq input boolean; LgrstOpenRtMdReq input boolean; INTMRSrcReqTp input Enum: SrcReqTp1; LgrstCloseLtSrcReqTp input Enum: SrcReqTp1; LgrstCloseRtSrcReqTp input Enum: SrcReqTp1; LgrstOpenLtSrcReqTp input Enum: SrcReqTp1; LgrstOpenRtSrcReqTp input Enum: SrcReqTp1; isINTMRDoneFailed input boolean; isLgrstCloseLDoneFailed input boolean; isLgrstCloseRDoneFailed input boolean; isLgrstOpenLDoneFailed input boolean; isLgrstOpenRDoneFailed input boolean; isINTMRDoneOK input boolean; isLgrstCloseLDoneOK input boolean; isLgrstCloseRDoneOK input boolean; isLgrstOpenLDoneOK input boolean; isLgrstOpenRDoneOK input boolean; SoftIntINTMR input boolean; SoftIntLgrstCloseLt input boolean; SoftIntLgrstCloseRt input boolean; SoftIntLgrstOpenLt input boolean; SoftIntLgrstOpenRt input boolean; SwIntINTMR input boolean; SwIntLgrstCloseLt input boolean; SwIntLgrstCloseRt input boolean; SwIntLgrstOpenLt input boolean; SwIntLgrstOpenRt input boolean; ModeSrcTpLgrstOpenL output Enum: SrcReqTp1; ModeSrcTpLgrstCloseL output Enum: SrcReqTp1; ModeSrcTpLgrstOpenR output Enum: SrcReqTp1; ModeSrcTpLgrstCloseR output Enum: SrcReqTp1; ModeSrcTpINTMR output Enum: SrcReqTp1; oModeRspLgrstOpenL output Enum: MdRspLocal1; oModeRspLgrstCloseL output Enum: MdRspLocal1; oModeRspLgrstOpenR output Enum: MdRspLocal1; oModeRspLgrstCloseR output Enum: MdRspLocal1; oModeRspINTMR output Enum: MdRspLocal1; LgrstOpenLBsy output boolean; LgrstCloseLBsy output boolean; LgrstOpenRBsy output boolean; LgrstCloseRBsy output boolean; INTMRBsy output boolean; is7s input boolean; is6s input boolean; is4s input boolean
  events: event input FUNCTION_CALL_EVENT

== stateflow chart ModeStatAndRsp/ModeStatAndRsp_Runnable_sys/Subsystem1/SRSModeCheck/Chart ==
  (default) -> (junction 5) : {i=0;}
  (junction 7) -> (junction 10) [order 1] : [Md_En[i] ==1&&MdSrcTp[i] ==SrcReqTp1.SrcReqTp_SRS]
  (junction 5) -> (junction 7) [order 1] : [i<ModeNum]
  (junction 7) -> (junction 16) [order 2]
  (junction 10) -> (junction 12) : {
      | U8SRSMode=i+1;
      | }
  (junction 16) -> (junction 5) : {i=i+1;}
  (junction 5) -> (junction 14) [order 2] : {
      | U8SRSMode=0;
      | }
  (junction 12) -> (junction 14)
  (junction 14) -> (junction 20)
  data: i local uint8; Md_En input boolean size=20; MdSrcTp input Enum: SrcReqTp1 size=20; U8SRSMode output uint8; ModeNum input uint8

== stateflow chart ModeStatAndRsp/ModeStatAndRsp_Runnable_sys/Subsystem1/FeedbackModeStatAndRsp/Chime2_3A6/Chart ==
  state CheckStat
    en:retrycnt=0;
    state Idle
      en:
      oChime = EventSts1.EventSts_NoAct;
    state Active1
      en:
      oChime = EventSts1.EventSts_Act;
    (default) -> CheckStat.Idle
    Active1 -> CheckStat.Idle [order 2] : [iChmMgrStat==2725||...
        | iChmMgrStat==0]
    Active1 -> CheckStat.Idle [order 1] : [after(ChmReqDurnTm/10,tick)]
        | {retrycnt=retrycnt+1;}
    CheckStat.Idle -> Active1 : [iChmMgrStat !=0&&iChmMgrStat!=2725&&retrycnt<4&&after(ChmReqIntlTm/10,tick)]
  state Idle
    en:
    oChime = EventSts1.EventSts_NoAct;
  state Cancel
    en:oChime = EventSts1.EventSts_CancleChime;
  state CancelwithNoCancel
    en:oChime = EventSts1.EventSts_NoAct;
  note: $0=NO_ACTION; $1=ACTIVE; $2=CANCEL_CHIME
  CheckStat -> CheckStat [order 3] : [hasChanged(iChmMgrStat)&&iChmMgrStat!=0&&iChmMgrStat!=2725]
  (default) -> Idle
  Idle -> CheckStat : [iChimActive]
  Cancel -> Idle : [after(ChmReqDurnTm/10,tick)]
  CheckStat -> Cancel [order 1] : [!iChimActive&&iChmMgrStat==2725]
  CancelwithNoCancel -> Cancel [order 2] : [iChmMgrStat==2725]
  CancelwithNoCancel -> Idle [order 1] : [after(ChmReqDurnTm/10,tick)]
  CheckStat -> CancelwithNoCancel [order 2] : [!iChimActive]
  data: iChmMgrStat input; iChimActive input boolean; oChime output Enum: EventSts1; retrycnt local uint8; ChmReqDurnTm input uint8; ChmReqIntlTm input uint8

== stateflow chart ModeStatAndRsp/ModeStatAndRsp_Runnable_sys/Subsystem1/Subsystem/Chart2 ==
  (default) -> (junction 3) : {ModeState32 = 0x00000000;}
  (junction 3) -> (junction 9) : {i = 0;}
  (junction 9) -> (junction 4) [order 1] : [i < 32]
  (junction 4) -> (junction 1) : {
      | temp_var = uint32(ModeArray[i]);
      | temp_var= temp_var << i;
      | ModeState32 = ModeState32 |  temp_var;
      | }
  (junction 1) -> (junction 9) : {i++;}
  (junction 9) -> (junction 5) [order 2]
  data: ModeState32 output uint32; ModeArray input boolean size=32; temp_var local uint32; i local uint8
